simulink model "Practica_4_simulink"  (R2024a)
settings: Solver=VariableStepAuto  StartTime=0.0  StopTime=10.0  RelTol=1e-3
InitFcn:
  | m=100;
  | r=0.05;
  | k=100;

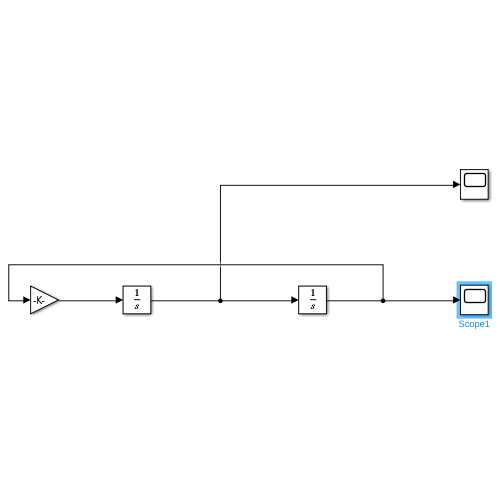
[thumbnail: Simulink's stored preview of the top-level diagram]
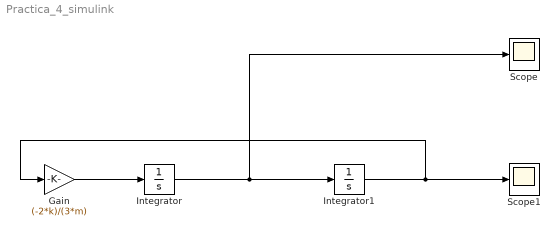
== system Practica_4_simulink ==
  Gain : Gain  Gain=(-2*k)/(3*m)
  Integrator : Integrator  InitialCondition=2
  Integrator1 : Integrator
  Scope : Scope
  Scope1 : Scope
  wires:
  Integrator/1 -> Scope/1, Integrator1/1
  Gain/1 -> Integrator/1
  Integrator1/1 -> Gain/1, Scope1/1
